simulink model "quadruple-tank-model"  (R2023b)
settings: Solver=VariableStepAuto  StartTime=0.0  StopTime=3000  RelTol=1e-3
undefined symbols (not defined in the file): A, A1, a1, a2, A2, a3, A3, A4, a4, B, C, D, g, initial_conditions, k1, k2, landa1, landa2, V1, V2
settings Model: Creator=Asus  LastModifiedBy=Asus

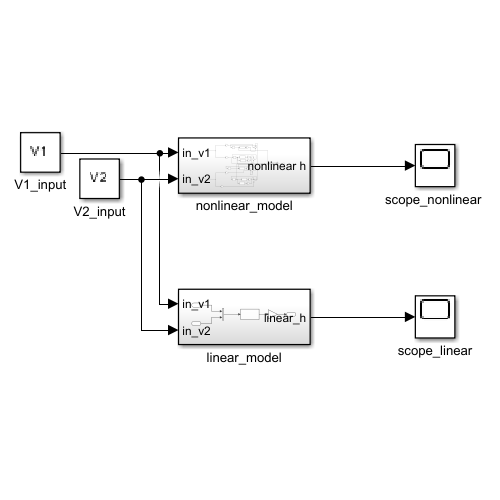
[thumbnail: Simulink's stored preview of the top-level diagram]
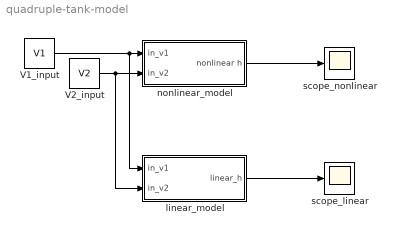
== system quadruple-tank-model ==
  V1_input : Constant  Value=V1
  V2_input : Constant  Value=V2
  linear_model : Subsystem
  nonlinear_model : Subsystem
  scope_linear : Scope
  "scope_nonlinear " : Scope
  wires:
  V1_input/1 -> linear_model/1(in_v1), nonlinear_model/1(in_v1)
  V2_input/1 -> nonlinear_model/2(in_v2), linear_model/2(in_v2)
  nonlinear_model/1(nonlinear h) -> "scope_nonlinear "/1
  linear_model/1(linear_h) -> scope_linear/1

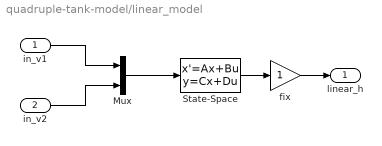
== system quadruple-tank-model/linear_model ==
  in_v1 : Inport
  in_v2 : Inport  Port=2
  Mux : Mux  Inputs=2
  State-Space : StateSpace  A=A  B=B  C=C  D=D  InitialCondition=initial_conditions
  fix : Gain
  linear_h : Outport
  wires:
  in_v1/1 -> Mux/1
  in_v2/1 -> Mux/2
  Mux/1 -> State-Space/1
  State-Space/1 -> fix/1
  fix/1 -> linear_h/1

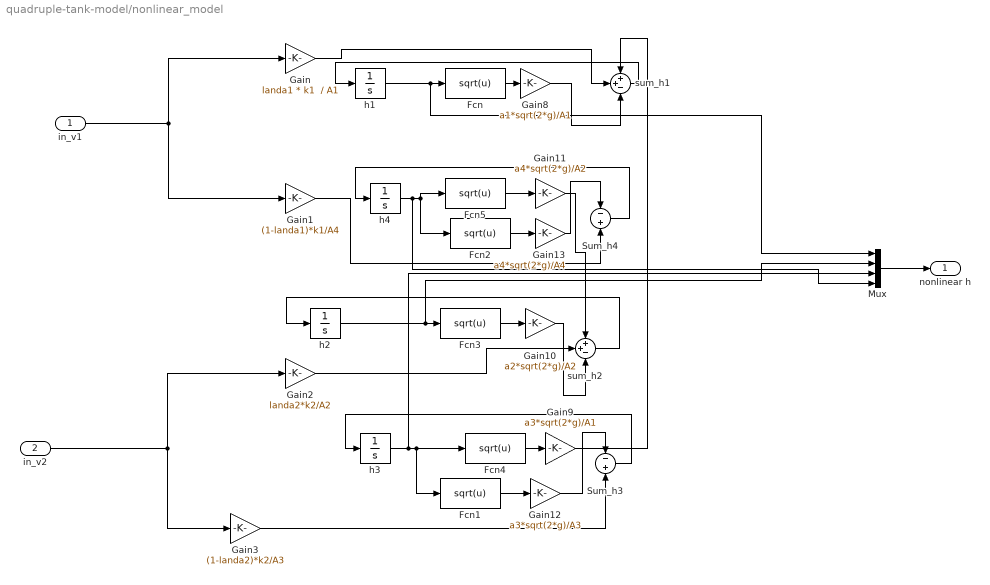
== system quadruple-tank-model/nonlinear_model ==
  in_v1 : Inport
  in_v2 : Inport  Port=2
  Fcn{,1..5} (6 alike) : Fcn  Expr=sqrt(u)
  Gain : Gain  Gain="landa1 * k1  / A1"
  Gain1 : Gain  Gain=(1-landa1)*k1/A4
  Gain10 : Gain  Gain=a2*sqrt(2*g)/A2
  Gain11 : Gain  Gain=a4*sqrt(2*g)/A2
  Gain12 : Gain  Gain=a3*sqrt(2*g)/A3
  Gain13 : Gain  Gain=a4*sqrt(2*g)/A4
  Gain2 : Gain  Gain=landa2*k2/A2
  Gain3 : Gain  Gain=(1-landa2)*k2/A3
  Gain8 : Gain  Gain=a1*sqrt(2*g)/A1
  Gain9 : Gain  Gain=a3*sqrt(2*g)/A1
  Mux : Mux
  Sum_h3 : Sum  Inputs=-+
  Sum_h4 : Sum  Inputs=-+
  h1 : Integrator  InitialCondition=initial_conditions(1)
  h2 : Integrator  InitialCondition=initial_conditions(2)
  h3 : Integrator  InitialCondition=initial_conditions(3)
  h4 : Integrator  InitialCondition=initial_conditions(4)
  sum_h1 : Sum  Inputs=++-
  sum_h2 : Sum  Inputs=++-
  nonlinear h : Outport
  wires:
  Gain12/1 -> Sum_h3/1
  Fcn3/1 -> Gain10/1
  h2/1 -> Mux/2, Fcn3/1
  Mux/1 -> nonlinear h/1
  Sum_h3/1 -> h3/1
  Gain9/1 -> sum_h1/1
  Fcn4/1 -> Gain9/1
  Gain2/1 -> sum_h2/2
  Fcn/1 -> Gain8/1
  Gain8/1 -> sum_h1/3
  h4/1 -> Mux/4, Fcn2/1, Fcn5/1
  Fcn1/1 -> Gain12/1
  sum_h2/1 -> h2/1
  Fcn5/1 -> Gain11/1
  in_v2/1 -> Gain3/1, Gain2/1
  Gain/1 -> sum_h1/2
  Sum_h4/1 -> h4/1
  Gain3/1 -> Sum_h3/2
  sum_h1/1 -> h1/1
  Gain1/1 -> Sum_h4/2
  h3/1 -> Mux/3, Fcn1/1, Fcn4/1
  Fcn2/1 -> Gain13/1
  h1/1 -> Mux/1, Fcn/1
  Gain10/1 -> sum_h2/3
  in_v1/1 -> Gain/1, Gain1/1
  Gain13/1 -> Sum_h4/1
  Gain11/1 -> sum_h2/1
